simulink model "ComplexTherma_Test_IGBT_Revised"  (R2017b)
settings: Solver=ode45  StartTime=0.0  StopTime=time  RelTol=1e-3  EnableMultiTasking=on
undefined symbols (not defined in the file or in its folder): vehicle_weight
libraries: powerlib x17
settings Model: Creator=fengqi.chang  LastModifiedBy=fengqi.chang
settings DataIOCC: LimitDataPoints=on  SaveFormat=Array
settings OptimizationCC: LifeSpan=inf
settings DebuggingCC: SolverPrmCheckMsg=warning  SFUnexpectedBacktrackingDiag=warning  SFNoUnconditionalDefaultTransitionDiag=warning  SFExecutionAtInitializationDiag=none
settings HardwareCC: ProdBitPerPointer=32  ProdBitPerSizeT=32  ProdBitPerPtrDiffT=32  ProdLargestAtomicFloat=None  ProdIntDivRoundTo=Undefined  ProdEndianess=Unspecified  ProdWordSize=32  ProdHWDeviceType=32-bit Generic
settings ModelReferenceCC: PropagateSignalLabelsOutOfModel=off
settings CodeAppCC: StateflowObjectComments=on
settings GRTTargetCC: TargetLangStandard=C89/C90 (ANSI)  GeneratePreprocessorConditionals=Disable all
settings ConfigComp: CovMetricSettings=dw  CovHtmlReporting=on  CovSaveCumulativeToWorkspaceVar=on  CovSaveSingleToWorkspaceVar=on  CovExternalEMLEnable=off  CovSFcnEnable=off
settings SimscapeCC: SimscapeNormalizeSystem=off

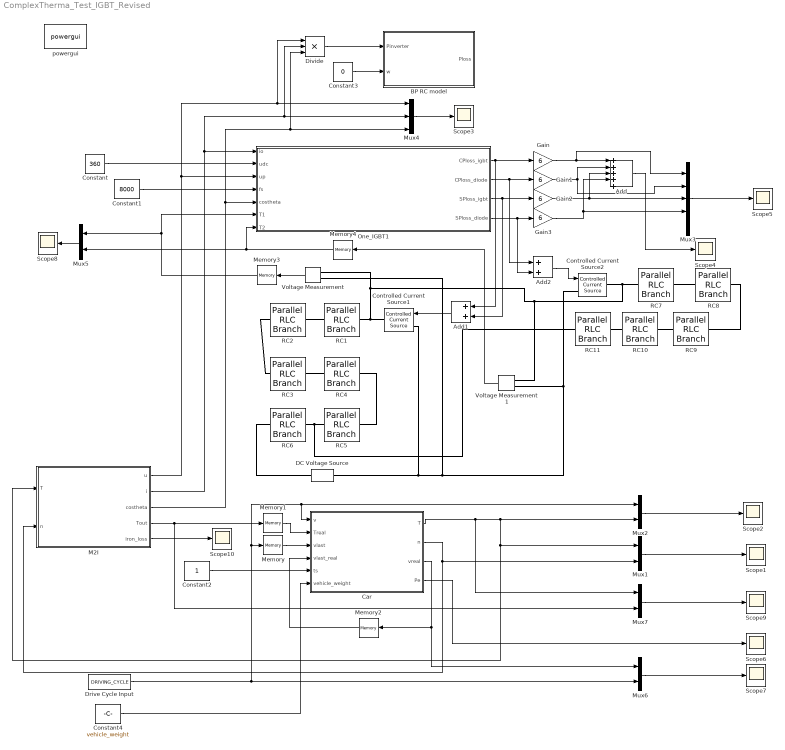
== system ComplexTherma_Test_IGBT_Revised ==
  Add : Sum  Inputs=+++++
  Add1 : Sum
  Add2 : Sum
  BP RC model : MATLAB Function  TreatAsAtomicUnit=on
  Car : MATLAB Function  TreatAsAtomicUnit=on
  Constant : Constant  Value=360
  Constant1 : Constant  Value=8000
  Constant2 : Constant
  Constant3 : Constant  Value=0
  Constant4 : Constant  Value=vehicle_weight
  Controlled Current Source1 : powerlib/Electrical Sources/Controlled Current Source  Initialize=on  Source_Type=AC  Amplitude=0  Phase=0  Frequency=0  Measurements=None
  Controlled Current Source2 : powerlib/Electrical Sources/Controlled Current Source  Initialize=on  Source_Type=AC  Amplitude=0  Phase=0  Frequency=0  Measurements=None
  DC Voltage Source : powerlib/Electrical Sources/DC Voltage Source  Amplitude=50  Measurements=None
  Divide : Product  Inputs=***
  Drive Cycle Input : FromWorkspace  VariableName=DRIVING_CYCLE  OutputAfterFinalValue=Setting to zero
  Gain{,1..3} (4 alike) : Gain  Gain=6
  M2I : MATLAB Function  TreatAsAtomicUnit=on
  Memory : Memory  InheritSampleTime=on
  Memory1 : Memory  InheritSampleTime=on
  Memory2 : Memory  InheritSampleTime=on
  Memory3 : Memory  InitialCondition=25  InheritSampleTime=on
  Memory4 : Memory  InitialCondition=25  InheritSampleTime=on
  Mux{1..2,5..7} (5 alike) : Mux  Inputs=2
  Mux3 : Mux  Inputs=5
  Mux4 : Mux  Inputs=3
  One_IGBT1 : MATLAB Function  TreatAsAtomicUnit=on
  RC1 : powerlib/Elements/Parallel RLC Branch  LConnTagsString=a  RConnTagsString=__new0  BranchType=RC  Resistance=0.0062  Inductance=1e-3  SetiL0=off  InitialCurrent=0  Capacitance=0.080645  Setx0=off  InitialVoltage=0  Measurements=None
  RC10 : powerlib/Elements/Parallel RLC Branch  LConnTagsString=a  RConnTagsString=__new0  BranchType=RC  Resistance=0.0331  Inductance=1e-3  SetiL0=off  InitialCurrent=0  Capacitance=11.78248  Setx0=off  InitialVoltage=0  Measurements=None
  RC11 : powerlib/Elements/Parallel RLC Branch  LConnTagsString=a  RConnTagsString=__new0  BranchType=RC  Resistance=0.0135  Inductance=1e-3  SetiL0=off  InitialCurrent=0  Capacitance=237.037  Setx0=off  InitialVoltage=0  Measurements=None
  RC2 : powerlib/Elements/Parallel RLC Branch  LConnTagsString=a  RConnTagsString=__new0  BranchType=RC  Resistance=0.022  Inductance=1e-3  SetiL0=off  InitialCurrent=0  Capacitance=0.909091  Setx0=off  InitialVoltage=0  Measurements=None
  RC3 : powerlib/Elements/Parallel RLC Branch  LConnTagsString=a  RConnTagsString=__new0  BranchType=RC  Resistance=0.0238  Inductance=1e-3  SetiL0=off  InitialCurrent=0  Capacitance=2.436975  Setx0=off  InitialVoltage=0  Measurements=None
  RC4 : powerlib/Elements/Parallel RLC Branch  LConnTagsString=a  RConnTagsString=__new0  BranchType=RC  Resistance=0.038  Inductance=1e-3  SetiL0=off  InitialCurrent=0  Capacitance=11.84211  Setx0=off  InitialVoltage=0  Measurements=None
  RC5 : powerlib/Elements/Parallel RLC Branch  LConnTagsString=a  RConnTagsString=__new0  BranchType=RC  Resistance=0.01  Inductance=1e-3  SetiL0=off  InitialCurrent=0  Capacitance=219  Setx0=off  InitialVoltage=0  Measurements=None
  RC6 : powerlib/Elements/Parallel RLC Branch  LConnTagsString=a  RConnTagsString=__new0  BranchType=R  Resistance=0.1  Inductance=1e-3  SetiL0=off  InitialCurrent=0  Capacitance=175  Setx0=on  InitialVoltage=0  Measurements=None
  RC7 : powerlib/Elements/Parallel RLC Branch  LConnTagsString=a  RConnTagsString=__new0  BranchType=RC  Resistance=0.0126  Inductance=1e-3  SetiL0=off  InitialCurrent=0  Capacitance=0.047619  Setx0=off  InitialVoltage=0  Measurements=None
  RC8 : powerlib/Elements/Parallel RLC Branch  LConnTagsString=a  RConnTagsString=__new0  BranchType=RC  Resistance=0.0391  Inductance=1e-3  SetiL0=off  InitialCurrent=0  Capacitance=0.434783  Setx0=off  InitialVoltage=0  Measurements=None
  RC9 : powerlib/Elements/Parallel RLC Branch  LConnTagsString=a  RConnTagsString=__new0  BranchType=RC  Resistance=0.0417  Inductance=1e-3  SetiL0=off  InitialCurrent=0  Capacitance=1.270983  Setx0=off  InitialVoltage=0  Measurements=None
  Scope{1..10} (10 alike) : Scope
  Voltage Measurement : powerlib/Measurements/Voltage Measurement  PhasorSimulation=off  OutputType=Complex  PSBequivalent=0
  Voltage Measurement1 : powerlib/Measurements/Voltage Measurement  PhasorSimulation=off  OutputType=Complex  PSBequivalent=0
  powergui : powerlib/powergui  Priority=1  SimulationMode=Discrete  SampleTime=1  frequency=60  Iterations=50  frequencyindice=0  Pbase=100e6  ErrMax=1e-4  UnitsV=kV  UnitsW=MW  buscounter=0  FunctionMessages=off  echomessages=off  EnableUseOfTLC=off  CurrentSourceSwitches=off  DisableSnubberDevices=off  DisableRonSwitches=off  DisableVfSwitches=off  DisplayEquations=off  SolverType=Backward Euler  Interpol=off  ExternalGateDelay=off  methode=off  Ts=100  x0status=blocks  SPID=off  SwTol=0  HookPort=off  RestoreLinks=warning  ResistiveCurrentMeasurement=off  Frange=[0:2:500]  Ylog=off  Xlog=on  ShowGrid=off  save=off  variable=ZData  structure=0  ZoomFFT=off  StartTime=0.0  cycles=1  DisplayStyle=1  fundamental=60  FreqAxis=off  MaxFrequency=1000  frequencyindicesteady=1  RmsSteady=1  display=off
  wires:
  Car/1(T) -> Mux7/1, M2I/1(T), Mux1/1, Mux2/2
  Car/2(n) -> M2I/2(n), Mux1/2
  Car/3(vreal) -> Mux6/1, Memory2/1
  M2I/3(costheta) -> One_IGBT1/5(costheta), Divide/3, Mux4/3
  Constant/1 -> One_IGBT1/2(udc)
  Constant1/1 -> One_IGBT1/4(fs)
  One_IGBT1/1(CPloss_igbt) -> Add1/1, Gain/1
  One_IGBT1/2(CPloss_diode) -> Add2/1, Gain1/1
  One_IGBT1/3(SPloss_igbt) -> Add1/2, Gain2/1
  One_IGBT1/4(SPloss_diode) -> Add2/2, Gain3/1
  Constant2/1 -> Car/5(ts)
  Gain/1 -> Mux3/1, Add/1
  Gain1/1 -> Mux3/2, Add/2
  Gain2/1 -> Mux3/3, Add/3
  Gain3/1 -> Add/4, Mux3/4
  Drive Cycle Input/1 -> Memory/1, Car/1(v), Mux2/1, Mux6/2
  M2I/4(Tout) -> Mux7/2, Memory1/1
  M2I/1(u) -> Divide/1, Mux4/1, One_IGBT1/3(up)
  Mux1/1 -> Scope1/1
  Memory1/1 -> Car/2(Treal)
  Mux2/1 -> Scope2/1
  Memory/1 -> Car/3(vlast)
  Memory2/1 -> Car/4(vlast_real)
  M2I/2(i) -> Divide/2, Mux4/2, One_IGBT1/1(io)
  Car/4(Pe) -> Scope6/1
  Add/1 -> Scope4/1
  Mux3/1 -> Scope5/1
  Mux4/1 -> Scope3/1
  Add1/1 -> Controlled Current Source1/1
  Voltage Measurement/1 -> Memory3/1
  Memory3/1 -> Mux5/1, One_IGBT1/6(T1)
  Add2/1 -> Controlled Current Source2/1
  Voltage Measurement1/1 -> Memory4/1
  Memory4/1 -> One_IGBT1/7(T2), Mux5/2
  Mux5/1 -> Scope8/1
  Constant3/1 -> BP RC model/2(w)
  Divide/1 -> BP RC model/1(Pinverter)
  Mux6/1 -> Scope7/1
  Mux7/1 -> Scope9/1
  M2I/5(iron_loss) -> Scope10/1
  Constant4/1 -> Car/6(vehicle_weight)
  connections:
  RC7/RConn1 -- Voltage Measurement/LConn1 -- RC1/RConn1 -- Controlled Current Source1/RConn1 -- Voltage Measurement1/LConn1 -- Controlled Current Source2/RConn1
  RC2/RConn1 -- RC1/LConn1
  RC2/LConn1 -- RC3/LConn1
  RC4/LConn1 -- RC3/RConn1
  RC4/RConn1 -- RC5/RConn1
  DC Voltage Source/RConn1 -- RC6/LConn1
  DC Voltage Source/LConn1 -- Controlled Current Source2/LConn1 -- Voltage Measurement1/LConn2 -- Voltage Measurement/LConn2 -- Controlled Current Source1/LConn1
  RC7/LConn1 -- RC8/RConn1
  RC8/LConn1 -- RC9/LConn1
  RC10/LConn1 -- RC9/RConn1
  RC11/LConn1 -- RC10/RConn1
  RC6/RConn1 -- RC11/RConn1 -- RC5/LConn1

== matlab function ComplexTherma_Test_IGBT_Revised/M2I ==
  data: T input; n input; u output; i output; costheta output; Tout output; iron_loss output
function [u,i,costheta,Tout,iron_loss] = PMSM2Inverter_Pcalc(T,n)
%%%%%%%%%%%%%%%%%%%%%%%Variable Table%%%%%%%%%%%%%%%%%%%%%%%%%%%%
%u          SQRT(3/2)*peak value of the output phase voltage from inverter    (V)
%i          SQRT(3/2)*peak value of the output phase current from inverter    (A)
%costheta   power factor required by the motor                      (none)
%T          torque required by the car                              (Nm)
%n          rotation speed of the motor required by the car         (rpm)
%%%%%%%%%%%%%%%%%%%%%%%%%%%%%%%%%%%%%%%%%%%%%%%%%%%%%%%%%%%%%%%%%
%%created in 2016 02 01 10 29
%%the model defines the interface of motor to inverter, which calculates 
%%the current, voltage as well as the power factor required by a motor.  
%%this model ignores the electrical transient status of the motor, but the
%%error caused is unclear yet.
%%this model is only valid for induction motor. For more complex ones,
%%model should be revised. 
%%%%%%%%%%%%%%%%%%%%%%%%Parameters%%%%%%%%%%%%%%%%%%%%%%%%%%%%%%%
Lq=8.0955e-5;
Ld=7.0955e-5;
p=6;%pair of polars
R=0.009;%resistor on stator, ohm%%%
psyr=0.05345836;%rotor permanent flux, Vs%%%
irate=450;%rated stator current, A, phase rms value
urate=160.1;%rated stator voltage, V, phase rms value
Prate=125000;%rated machinery power, W,
%%%%%%%%%%%%%%%%%%input preparation%%%%%%%%%%%%%%%%%%%%
wr=n*p/60*2*pi;
isq=T/p/psyr;
isd=0;
usd=-Lq*isq*wr+R*isd;
usq=(Ld*isd+psyr)*wr+R*isq;

i=sqrt(isq*isq+isd*isd);
u=sqrt(usq*usq+usd*usd);
costheta=(usd*isd+usq*isq)/u/i;%cos(atan(usq/usd)-atan(isq/isd));
Tout=T;
%%%%%%%%%%%%%if flux weakening required%%%%%%%%%%%%%%%%
if(u>(urate*sqrt(3)))
    if(abs(n*T*2*pi/60)>=Prate)
        Tout=Prate/(n/60*2*pi);
    else
        Tout=T;
    end
    psy_l=0;
    psy_h=psyr;
    psy_iter=(psy_l+psy_h)/2;
    u_iter=u;
    while(abs(urate*sqrt(3)-u_iter)>1)%iteration to calculate the right psy to reach urate
        isd=(psy_iter-psyr)/Ld;
        isq=T/(p*psyr+p*(Ld-Lq)*isd);
        usd=-Lq*isq*wr+R*isd;
        usq=(Ld*isd+psyr)*wr+R*isq;
        u=sqrt(usq*usq+usd*usd);
        u_iter=u;
        if(u_iter>urate*sqrt(3))
            psy_h=psy_iter;
            psy_iter=0.5*(psy_l+psy_h);
        else
            psy_l=psy_iter;
            psy_iter=0.5*(psy_l+psy_h);
        end
    end
    
end
i=sqrt(isq*isq+isd*isd);
u=sqrt(usq*usq+usd*usd);
costheta=(usd*isd+usq*isq)/u/i;%cos(atan(usq/usd)-atan(isq/isd));
% if(i>(irate*sqrt(3)))
%     isq=isq*irate*1.414/i;%no max torque algorithm is applied
%     isd=isd*irate*1.414/i;
%     Tout=isq*p/Lr*Lm*isd*Lm;
%     wsl=Tout/p*Rr/(Lm*isd)^2;
%     wk=wsl+n*p/60*2*pi;
%     usd=Rs*isd-wk*(Ls*isq+Lm*(-isq*Lm/Lr));
%     usq=Rs*isq+wk*Ls*isd;
%     i=sqrt(isq*isq+isd*isd);%
%     u=sqrt(usq*usq+usd*usd);
% end
%iron_loss = (9.128008725474993e-06*n^2 + 0.119030169537619*n)/3.3007*(abs(T)^0.5186);
beta = [7.47991049806284e-06,-0.00164430283336243,0.152741302836017,0.945215242366288];
iron_loss = (beta(1).*n.^2 + beta(2).*n).*beta(3).*(abs(T).^beta(4));

if isnan(costheta)
    costheta=1;
end
if(n<0.1)&&(T==0)
    u=0;
    i=0;
    Tout=0;
    costheta=1;
end
if (Tout~=T)
    Tout=T;
end

== matlab function ComplexTherma_Test_IGBT_Revised/Car ==
  data: v input; T output; Treal input; vlast input; vlast_real input; ts input; n output; vreal output; Pe output; vehicle_weight input
function [T,n,vreal,Pe] = CarModel(v,Treal,vlast,vlast_real,ts,vehicle_weight)
%%%%%%%%%%%%%%%%%%%%%%%%%%%%varialbe table%%%%%%%%%%%%%%%%%%%%%%%%%%%%%%%%%
%variavle name      meaning,                                             unit
%a,                 acceleration order of the car,                       (m/s^2)
%v,                 speed order of the car,                              (m/s)
%T,                 torque of the motor required by the car,             (Nm)
%n,                 rotation speed of the motor,                         (rpm)
%Pe,                power of the motor required by the car,              (kW)
%a_real,            real acceleration of the car,                        (m/s^2)
%vlast,             real speed of the car in last simulation period,     (m/s)
%nlast,             real rotation speed of the motor in last period,     (rad/s)
%Treal,             real torque from motor in  last simulation period,   (Nm)
%vnext,             real speed of the car,                               (m/s)
%ts,                simulation period,                                   (s)
%%%%%%%%%%%%%%%%%%%%%%%%%%%%%%%%%%%%%%%%%%%%%%%%%%%%%%%%%%%%%%%%%%%%%%%%%%%
%%%%%%%%%%%%%%%%%%%%%%%%%%%%parameter table%%%%%%%%%%%%%%%%%%%%%%%%%%%%%%%%
m=vehicle_weight;%1443.331;%1195;%                                  mass of the car,                      (kg)
yeta_t=0.98;%                             efficiency of the transmission,       ()

i_g=9.7;%                                 transmission ratio fo the driveline,  ()
R=0.350;%                                 radius of the tyre,                   (m)


a=(v-vlast)/ts;%calculate the acceleration needed in the next simulation period
if (vlast==0)&&(a==0)
    T=0;
else
    T = 1/yeta_t*(105.0138054720000+6.602356610980250*(vlast+v)/2+0.260513017636277*(vlast^2+v^2)/2+m*a)/(1/R*i_g);
    %parameters obtained from Agonne National Lab Testing Report
end
if (vlast==0)&&(Treal==0)
    areal=0;
else
    areal=(Treal*1/R*i_g*yeta_t-105.0138054720000-6.602356610980250*(vlast+v)/2-0.260513017636277*(vlast^2+v^2)/2)/(m);%calculate the real acceleration using Treal provided by the last simulation period
end
if(T<=0)&&(vlast_real<=0)
    T=0;
    areal=0;
end
vreal=vlast_real+areal*ts;%calculate the real speed in the next simulation period
n=(v+vlast)/2/R*i_g*30/pi;%calculate the real rotation speed in the next simulation period, in rpm
Pe=n*T/60*2*pi;%calculate the power needed in the next simulation period
end

== matlab function ComplexTherma_Test_IGBT_Revised/BP RC model ==
  data: Pinverter input; Ploss output; w input
function Ploss = BatteryPack_RC_model(Pinverter,w)
%%%%%%%%%%%%%%%%%%%%%%%%%%%%%%%%%%%%%%%
%This is the model to test the impact of different cutrrent waveforms on
%battery pack
%The voltage and capacity is configurable
upack=380;%the voltage of battery pack
parallel=1;%The number divided by parallel
series=1;%The number divided by series connection
i=(Pinverter/parallel)/(upack/series);%calculate the current of the module
w=w*2;%w is the frequency of the DC bus current
RC_up=complex(0.0608*6.75,0.051*6.75*w)*parallel/series;
RC_dw=complex(120,120*1.2571*w);
%%%%%%%%%%%%%%%%%%%%%%%%%%%%%%%%%%%%%%%%
%RC_up and RC_dw are the resistance function of the battery pack
U=i*RC_up/RC_dw;
Pmodule=real(i*U);
Ploss=Pmodule*parallel*series;

== matlab function ComplexTherma_Test_IGBT_Revised/One_IGBT1 ==
  data: io input; udc input; up input; fs input; CPloss_igbt output; CPloss_diode output; costheta input; SPloss_igbt output; SPloss_diode output; T1 input; T2 input
%%created in 2016 01 31 15 42
%%the model defines the input and output of the loss model of one switch
%%that is only the simplest version of an IGBT model
function [CPloss_igbt,CPloss_diode,SPloss_igbt,SPloss_diode] = IGBT_FS800R07A2E3(io,udc,up,fs,costheta,T1,T2)
%%this model is only for voltage source inverter or converter
%%%%%%%%%%%%%%%%%%%%%%%%%%%%parameter table%%%%%%%%%%%%%%%%%%%%%%%%%%%%%%%%
%%%%%%%%%%%%%%%%%%%%%%%%%%%%varialbe table%%%%%%%%%%%%%%%%%%%%%%%%%%%%%%%%%
%variavle name      meaning,                                                        unit
%io,                operation current, sqrt(3/2) peak value of phase current,       (A)
%up,                operation voltage, sqrt(3/2) peak value of phase voltage,       (V)
%udc,               DC bus voltage,                                                 (V)
%fs,                switching frequency,                                            (Hz)
%costheta,          power factor,                                                   (none)
%CPloss_igbt,       conduction loss on IGBT,                                        (W)
%CPloss_diode,      conduction loss on the reverse paralleled diode,                (W)
%SPloss_igbt,       switching loss on IGBT,                                         (W)
%SPloss_diode,      switching loss on the reverse paralleled diode,                 (W)
%%%%%%%%%%%%%%%%%%%%%%%%%%%%%%%%%%%%%%%%%%%%%%%%%%%%%%%%%%%%%%%%%%%%%%%%%%%
io=io/sqrt(3/2);
% uce=0.75-0.002*(T1-25);%@25degree, @150degress is 1.98V
% rc=0.85/600*(1+0.0052427*(T1-25));%
% udsat=0.8-0.002*(T2-25) ;%
% rd=0.6/400*(1+0.002*(T2-25));%

rc = 0.9/900*(1 + 0.0045*(T1 - 25))/4*3;%0.9/900*(1+0.0052427*(T1 - 25));%resistor on the line and connection, usually ignored
rd = 0.6/400*(1 + 0.00167*(T2 - 25))/4*3;%0.6/400*(1+0.002*(T2 - 25));%resistor on the diode path, usually ignored
uce = 0.75 - 0.002*(T1 - 25);%0.75-0.002*(T1 - 25);%@25degree, @150degress is 1.98V
udsat = 0.8 - 0.002*(T2 - 25);%0.8-0.002*(T2 - 25);%

m=up/sqrt(3/2)*2/udc;%modulation index
Eon_igbt=(0.011+0.0085/350*(abs(io)/4*3*(2/pi)-400))*((T1-125)*0.00129+1)/3*4;% that is only the typical value, the value is influenced by T,r_gate and Ic
Eoff_igbt=(0.0175+0.0105/300*(abs(io)/4*3*(2/pi)-400))*((T1-125)*0.00148+1)/3*4;%that is only the typical value, the value is influenced by T,r_gate and Ic
Eon_diode=0;%that value is usually neglected
Eoff_diode=(0.007+0.0045/300*(abs(io)*(2/pi)/4*3-400))*((T2-125)*0.008571+1)/3*4;%that is only the typical value, the value is influenced by T,r_gate and Ic
CPloss_igbt=uce*abs(io)*(1/2/pi+m*costheta/8)+rc*io*io*(1/8+m*costheta/3/pi);
CPloss_diode=udsat*abs(io)*(1/2/pi-m*costheta/8)+rd*io*io*(1/8-m*costheta/3/pi);
SPloss_igbt=fs*(Eon_igbt+Eoff_igbt)/300*udc;
SPloss_diode=fs*(Eon_diode+Eoff_diode);
if(io==0)
    SPloss_igbt=0;
    SPloss_diode=0;
end
end
